simulink model "FS10"  (R2017a)
settings: Solver=VariableStepAuto  StartTime=0.0  StopTime=runtime  RelTol=1e-3
values from neighbouring files (symbols this model uses):
  C1 = [0.668571650540611,0.505734391442468,0.511990363346558,0.532740104446010,0.361957267040408,0.712570423425208,0.623515243156496,0.537105734466424,0.707123883207618,0.460578686491704]    [BaseTest.m]    (also in FStest10.m)
  C2 = [0.093600031075686,0.070802814801946,0.092158265402380,0.095893218800282,0.043434872044849,0.106885563513781,0.087292134041909,0.091307974859292,0.120211060145295,0.082904163568507]    [BaseTest.m]    (also in FStest10.m)
  dn = 0.5    [BaseTest.m]    (also in FStest10.m = 2)
  dncons = 7    [FStest10.m]
  IP = [117,104,91,78,65,52,39,26,13,0]    [BaseTest.m]    (also in FStest10.m)
  IV = 0    [BaseTest.m]    (also in FStest10.m)
  maxa = 1    [BaseTest.m]    (also in FStest10.m)
  maxv = 40    [BaseTest.m]    (also in FStest10.m)
  mina = -3    [BaseTest.m]    (also in FStest10.m)
  ring = 130    [BaseTest.m]    (also in FStest10.m)
  T = [82,96,76,78,94,117,83,100,91,111]    [BaseTest.m]    (also in FStest10.m)
  U = [0  2  2.5 3.0 3.2 3.4 3.4  4 0 0  ]    [FStest10.m]
  Ut = [0 220 240 260 280 320 400 10000 10001 10002]    [FStest10.m]
undefined symbols (not defined in the file or in its folder): DiscIntNeverNeededParam
libraries: visionstatistics x10, dspstat3 x10, powerlib_meascontrol x1
settings Model: Creator=ttal5  LastModifiedBy=ttal5

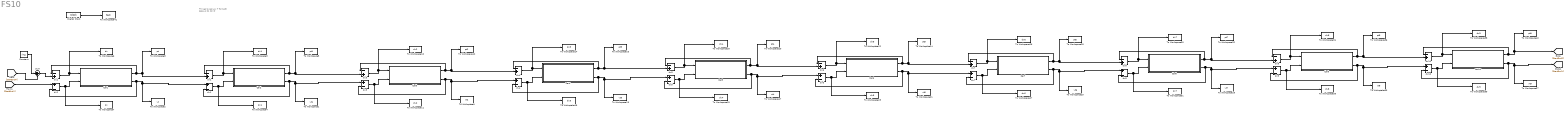
== system FS10 ==
  note: Things to set up:
      | T for both delays
      | C1
      | C2
      | IP
  Car1 : Subsystem
  Car10 : Subsystem
  Car2 : Subsystem
  Car3 : Subsystem
  Car4 : Subsystem
  Car5 : Subsystem
  Car6 : Subsystem
  Car7 : Subsystem
  Car8 : Subsystem
  Car9 : Subsystem
  Constant : Constant  Value=ring
  Digital Clock : DigitalClock  SampleTime=0.01
  Sum : Sum  Inputs=|++
  To Workspace1 : ToWorkspace  VariableName=vt1  SampleTime=0.01
  To Workspace10 : ToWorkspace  VariableName=dx2  SampleTime=0.01
  To Workspace11 : ToWorkspace  VariableName=dv2  SampleTime=0.01
  To Workspace12 : ToWorkspace  VariableName=pt2  SampleTime=0.01
  To Workspace13 : ToWorkspace  VariableName=vt3  SampleTime=0.01
  To Workspace14 : ToWorkspace  VariableName=dx3  SampleTime=0.01
  To Workspace15 : ToWorkspace  VariableName=dv3  SampleTime=0.01
  To Workspace16 : ToWorkspace  VariableName=pt3  SampleTime=0.01
  To Workspace17 : ToWorkspace  VariableName=vt4  SampleTime=0.01
  To Workspace18 : ToWorkspace  VariableName=dx4  SampleTime=0.01
  To Workspace19 : ToWorkspace  VariableName=dv4  SampleTime=0.01
  To Workspace2 : ToWorkspace  VariableName=vt  SampleTime=0.01
  To Workspace20 : ToWorkspace  VariableName=pt4  SampleTime=0.01
  To Workspace21 : ToWorkspace  VariableName=vt5  SampleTime=0.01
  To Workspace22 : ToWorkspace  VariableName=dx5  SampleTime=0.01
  To Workspace23 : ToWorkspace  VariableName=dv5  SampleTime=0.01
  To Workspace24 : ToWorkspace  VariableName=pt5  SampleTime=0.01
  To Workspace25 : ToWorkspace  VariableName=vt6  SampleTime=0.01
  To Workspace26 : ToWorkspace  VariableName=dx6  SampleTime=0.01
  To Workspace27 : ToWorkspace  VariableName=dv6  SampleTime=0.01
  To Workspace28 : ToWorkspace  VariableName=pt6  SampleTime=0.01
  To Workspace29 : ToWorkspace  VariableName=vt7  SampleTime=0.01
  To Workspace3 : ToWorkspace  VariableName=dx1  SampleTime=0.01
  To Workspace30 : ToWorkspace  VariableName=dx7  SampleTime=0.01
  To Workspace31 : ToWorkspace  VariableName=dv7  SampleTime=0.01
  To Workspace32 : ToWorkspace  VariableName=pt7  SampleTime=0.01
  To Workspace33 : ToWorkspace  VariableName=vt8  SampleTime=0.01
  To Workspace34 : ToWorkspace  VariableName=dx8  SampleTime=0.01
  To Workspace35 : ToWorkspace  VariableName=dv8  SampleTime=0.01
  To Workspace36 : ToWorkspace  VariableName=pt8  SampleTime=0.01
  To Workspace37 : ToWorkspace  VariableName=vt9  SampleTime=0.01
  To Workspace38 : ToWorkspace  VariableName=dx9  SampleTime=0.01
  To Workspace39 : ToWorkspace  VariableName=dv9  SampleTime=0.01
  To Workspace4 : ToWorkspace  VariableName=dv1  SampleTime=0.01
  To Workspace40 : ToWorkspace  VariableName=pt9  SampleTime=0.01
  To Workspace41 : ToWorkspace  VariableName=ttest  SampleTime=0.01
  To Workspace5 : ToWorkspace  VariableName=pt1  SampleTime=0.01
  To Workspace6 : ToWorkspace  VariableName=dx  SampleTime=0.01
  To Workspace7 : ToWorkspace  VariableName=dv  SampleTime=0.01
  To Workspace8 : ToWorkspace  VariableName=pt  SampleTime=0.01
  To Workspace9 : ToWorkspace  VariableName=vt2  SampleTime=0.01
  dv{1..10} (10 alike) : Sum  Inputs=+-
  dx{1..10} (10 alike) : Sum  Inputs=-+  OutMin=[0]
  wires:
  dv1/1 -> To Workspace4/1, Car2/2(dv)
  dx1/1 -> To Workspace3/1, Car2/1(dx)
  Car1/1(Pos1) -> dx2/1, dx1/2, To Workspace8/1
  Car1/2(Vel1) -> dv1/1, To Workspace2/1, dv2/2
  dv2/1 -> To Workspace7/1, Car1/2(dv)
  dx2/1 -> To Workspace6/1, Car1/1(dx)
  [StartEndP] -> Sum/2
  [StartEndV] -> dv2/1
  dv3/1 -> To Workspace11/1, Car3/2(dv)
  dx3/1 -> To Workspace10/1, Car3/1(dx)
  Car2/1(Pos1) -> dx1/1, dx3/2, To Workspace5/1
  Car2/2(Vel1) -> dv3/1, To Workspace1/1, dv1/2
  dv4/1 -> To Workspace15/1, Car4/2(dv)
  dx4/1 -> To Workspace14/1, Car4/1(dx)
  Car3/1(Pos1) -> dx3/1, dx4/2, To Workspace12/1
  Car3/2(Vel1) -> dv4/1, To Workspace9/1, dv3/2
  dv5/1 -> To Workspace19/1, Car5/2(dv)
  dx5/1 -> To Workspace18/1, Car5/1(dx)
  Car4/1(Pos1) -> dx4/1, dx5/2, To Workspace16/1
  Car4/2(Vel1) -> dv5/1, To Workspace13/1, dv4/2
  dv6/1 -> To Workspace23/1, Car6/2(dv)
  dx6/1 -> To Workspace22/1, Car6/1(dx)
  Car5/1(Pos1) -> dx5/1, dx6/2, To Workspace20/1
  Car5/2(Vel1) -> dv6/1, To Workspace17/1, dv5/2
  dv7/1 -> To Workspace27/1, Car7/2(dv)
  dx7/1 -> To Workspace26/1, Car7/1(dx)
  Car6/1(Pos1) -> dx6/1, dx7/2, To Workspace24/1
  Car6/2(Vel1) -> To Workspace21/1, dv7/1, dv6/2
  dv8/1 -> To Workspace31/1, Car8/2(dv)
  dx8/1 -> To Workspace30/1, Car8/1(dx)
  Car7/1(Pos1) -> dx7/1, dx8/2, To Workspace28/1
  Car7/2(Vel1) -> dv8/1, To Workspace25/1, dv7/2
  dv9/1 -> To Workspace35/1, Car9/2(dv)
  dx9/1 -> To Workspace34/1, Car9/1(dx)
  Car8/1(Pos1) -> dx8/1, dx9/2, To Workspace32/1
  Car8/2(Vel1) -> dv9/1, To Workspace29/1, dv8/2
  Car10/2(Vel1) -> [StartEndV], To Workspace37/1, dv10/2
  dv10/1 -> To Workspace39/1, Car10/2(dv)
  dx10/1 -> To Workspace38/1, Car10/1(dx)
  Car10/1(Pos1) -> dx10/1, [StartEndP], To Workspace40/1
  Car9/1(Pos1) -> dx9/1, dx10/2, To Workspace36/1
  Car9/2(Vel1) -> dv10/1, To Workspace33/1, dv9/2
  Constant/1 -> Sum/1
  Sum/1 -> dx2/2
  Digital Clock/1 -> To Workspace41/1

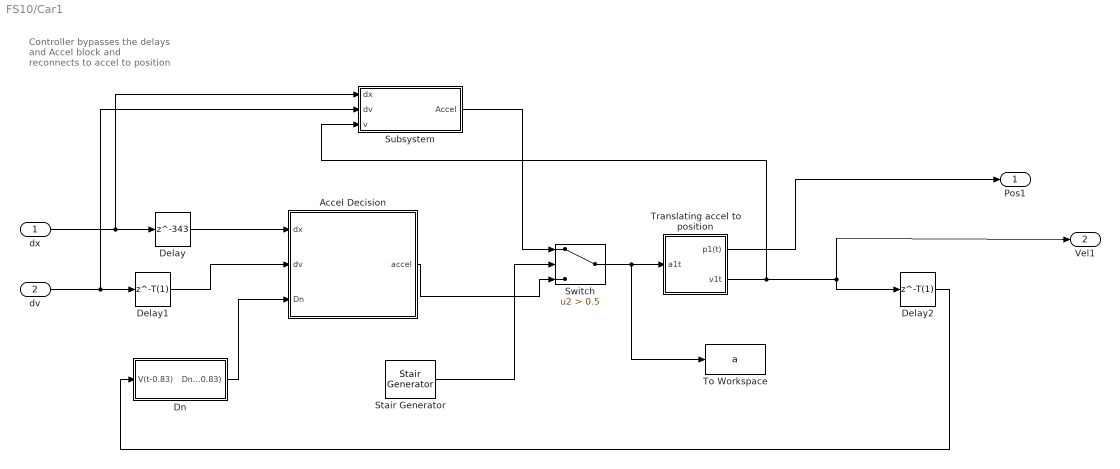
== system FS10/Car1 ==
  note: Controller bypasses the delays and Accel block and reconnects to accel to position
  dx : Inport
  dv : Inport  Port=2
  Accel Decision : Subsystem
  Delay : Delay  DelayLength=343  InitialCondition=IP(1)-IP(2)  SampleTime=0.01
  Delay1 : Delay  DelayLength=T(1)  SampleTime=0.01
  Delay2 : Delay  DelayLength=T(1)  SampleTime=0.01
  Dn : Subsystem
  Stair Generator : powerlib_meascontrol/Pulse & Signal Generators/Stair Generator  t=FStime  e=[0 1 1 0]  Ts=0.01
      settings: SourceProductName=Simscape Power Systems
  Subsystem : Subsystem
  Switch : Switch  Criteria=u2 > Threshold  Threshold=0.5
  To Workspace : ToWorkspace  VariableName=a  SampleTime=0.01
  Translating accel to position : Subsystem
  Pos1 : Outport
  Vel1 : Outport  Port=2
  wires:
  Translating accel to position/1(p1(t)) -> Pos1/1
  Delay/1 -> Accel Decision/1(dx)
  Accel Decision/1(accel) -> Switch/3
  Translating accel to position/2(v1t) -> Subsystem/3(v), Delay2/1, Vel1/1
  Delay2/1 -> Dn/1(V(t-0.83))
  Dn/1(Dn(t-0.83)) -> Accel Decision/3(Dn)
  Delay1/1 -> Accel Decision/2(dv)
  dx/1 -> Subsystem/1(dx), Delay/1
  dv/1 -> Subsystem/2("dv "), Delay1/1
  Subsystem/1(Accel) -> Switch/1
  Switch/1 -> To Workspace/1, Translating accel to position/1(a1t)
  Stair Generator/1 -> Switch/2

== system FS10/Car10 ==
  dx : Inport
  dv : Inport  Port=2
  Accel Decision : Subsystem
  Delay : Delay  DelayLength=343  InitialCondition=IP(1)-IP(2)  SampleTime=0.01
  Delay1 : Delay  DelayLength=T(10)  SampleTime=0.01
  Delay2 : Delay  DelayLength=T(10)  SampleTime=0.01
  Dn : Subsystem
  To Workspace : ToWorkspace  VariableName=a10  SampleTime=-1
  Translating accel to position : Subsystem
  Pos1 : Outport
  Vel1 : Outport  Port=2
  wires:
  Translating accel to position/1(p1(t)) -> Pos1/1
  Delay/1 -> Accel Decision/1(dx)
  Accel Decision/1(accel) -> To Workspace/1, Translating accel to position/1(a1t)
  Translating accel to position/2(v1t) -> Delay2/1, Vel1/1
  Delay2/1 -> Dn/1(V(t-0.83))
  Dn/1(Dn(t-0.83)) -> Accel Decision/3(Dn)
  Delay1/1 -> Accel Decision/2(dv)
  dx/1 -> Delay/1
  dv/1 -> Delay1/1

== system FS10/Car2 ==
  dx : Inport
  dv : Inport  Port=2
  Accel Decision : Subsystem
  Delay : Delay  DelayLength=343  InitialCondition=IP(1)-IP(2)  SampleTime=0.01
  Delay1 : Delay  DelayLength=T(2)  SampleTime=0.01
  Delay2 : Delay  DelayLength=T(2)  SampleTime=0.01
  Dn : Subsystem
  To Workspace : ToWorkspace  VariableName=a2  SampleTime=-1
  Translating accel to position : Subsystem
  Pos1 : Outport
  Vel1 : Outport  Port=2
  wires:
  Translating accel to position/1(p1(t)) -> Pos1/1
  Delay/1 -> Accel Decision/1(dx)
  Accel Decision/1(accel) -> To Workspace/1, Translating accel to position/1(a1t)
  Translating accel to position/2(v1t) -> Delay2/1, Vel1/1
  Delay2/1 -> Dn/1(V(t-0.83))
  Dn/1(Dn(t-0.83)) -> Accel Decision/3(Dn)
  Delay1/1 -> Accel Decision/2(dv)
  dx/1 -> Delay/1
  dv/1 -> Delay1/1

== system FS10/Car3 ==
  dx : Inport
  dv : Inport  Port=2
  Accel Decision : Subsystem
  Delay : Delay  DelayLength=343  InitialCondition=IP(1)-IP(2)  SampleTime=0.01
  Delay1 : Delay  DelayLength=T(3)  SampleTime=0.01
  Delay2 : Delay  DelayLength=T(3)  SampleTime=0.01
  Dn : Subsystem
  To Workspace : ToWorkspace  VariableName=a3  SampleTime=-1
  Translating accel to position : Subsystem
  Pos1 : Outport
  Vel1 : Outport  Port=2
  wires:
  Translating accel to position/1(p1(t)) -> Pos1/1
  Delay/1 -> Accel Decision/1(dx)
  Accel Decision/1(accel) -> To Workspace/1, Translating accel to position/1(a1t)
  Translating accel to position/2(v1t) -> Delay2/1, Vel1/1
  Delay2/1 -> Dn/1(V(t-0.83))
  Dn/1(Dn(t-0.83)) -> Accel Decision/3(Dn)
  Delay1/1 -> Accel Decision/2(dv)
  dx/1 -> Delay/1
  dv/1 -> Delay1/1

== system FS10/Car4 ==
  dx : Inport
  dv : Inport  Port=2
  Accel Decision : Subsystem
  Delay : Delay  DelayLength=343  InitialCondition=IP(1)-IP(2)  SampleTime=0.01
  Delay1 : Delay  DelayLength=T(4)  SampleTime=0.01
  Delay2 : Delay  DelayLength=T(4)  SampleTime=0.01
  Dn : Subsystem
  To Workspace : ToWorkspace  VariableName=a4  SampleTime=-1
  Translating accel to position : Subsystem
  Pos1 : Outport
  Vel1 : Outport  Port=2
  wires:
  Translating accel to position/1(p1(t)) -> Pos1/1
  Delay/1 -> Accel Decision/1(dx)
  Accel Decision/1(accel) -> To Workspace/1, Translating accel to position/1(a1t)
  Translating accel to position/2(v1t) -> Delay2/1, Vel1/1
  Delay2/1 -> Dn/1(V(t-0.83))
  Dn/1(Dn(t-0.83)) -> Accel Decision/3(Dn)
  Delay1/1 -> Accel Decision/2(dv)
  dx/1 -> Delay/1
  dv/1 -> Delay1/1

== system FS10/Car5 ==
  dx : Inport
  dv : Inport  Port=2
  Accel Decision : Subsystem
  Delay : Delay  DelayLength=343  InitialCondition=IP(1)-IP(2)  SampleTime=0.01
  Delay1 : Delay  DelayLength=T(5)  SampleTime=0.01
  Delay2 : Delay  DelayLength=T(5)  SampleTime=0.01
  Dn : Subsystem
  To Workspace : ToWorkspace  VariableName=a5  SampleTime=-1
  Translating accel to position : Subsystem
  Pos1 : Outport
  Vel1 : Outport  Port=2
  wires:
  Translating accel to position/1(p1(t)) -> Pos1/1
  Delay/1 -> Accel Decision/1(dx)
  Accel Decision/1(accel) -> To Workspace/1, Translating accel to position/1(a1t)
  Translating accel to position/2(v1t) -> Delay2/1, Vel1/1
  Delay2/1 -> Dn/1(V(t-0.83))
  Dn/1(Dn(t-0.83)) -> Accel Decision/3(Dn)
  Delay1/1 -> Accel Decision/2(dv)
  dx/1 -> Delay/1
  dv/1 -> Delay1/1

== system FS10/Car6 ==
  dx : Inport
  dv : Inport  Port=2
  Accel Decision : Subsystem
  Delay : Delay  DelayLength=343  InitialCondition=IP(1)-IP(2)  SampleTime=0.01
  Delay1 : Delay  DelayLength=T(6)  SampleTime=0.01
  Delay2 : Delay  DelayLength=T(6)  SampleTime=0.01
  Dn : Subsystem
  To Workspace : ToWorkspace  VariableName=a6  SampleTime=-1
  Translating accel to position : Subsystem
  Pos1 : Outport
  Vel1 : Outport  Port=2
  wires:
  Translating accel to position/1(p1(t)) -> Pos1/1
  Delay/1 -> Accel Decision/1(dx)
  Accel Decision/1(accel) -> To Workspace/1, Translating accel to position/1(a1t)
  Translating accel to position/2(v1t) -> Delay2/1, Vel1/1
  Delay2/1 -> Dn/1(V(t-0.83))
  Dn/1(Dn(t-0.83)) -> Accel Decision/3(Dn)
  Delay1/1 -> Accel Decision/2(dv)
  dx/1 -> Delay/1
  dv/1 -> Delay1/1

== system FS10/Car7 ==
  dx : Inport
  dv : Inport  Port=2
  Accel Decision : Subsystem
  Delay : Delay  DelayLength=343  InitialCondition=IP(1)-IP(2)  SampleTime=0.01
  Delay1 : Delay  DelayLength=T(7)  SampleTime=0.01
  Delay2 : Delay  DelayLength=T(7)  SampleTime=0.01
  Dn : Subsystem
  To Workspace : ToWorkspace  VariableName=a7  SampleTime=-1
  Translating accel to position : Subsystem
  Pos1 : Outport
  Vel1 : Outport  Port=2
  wires:
  Translating accel to position/1(p1(t)) -> Pos1/1
  Delay/1 -> Accel Decision/1(dx)
  Accel Decision/1(accel) -> To Workspace/1, Translating accel to position/1(a1t)
  Translating accel to position/2(v1t) -> Delay2/1, Vel1/1
  Delay2/1 -> Dn/1(V(t-0.83))
  Dn/1(Dn(t-0.83)) -> Accel Decision/3(Dn)
  Delay1/1 -> Accel Decision/2(dv)
  dx/1 -> Delay/1
  dv/1 -> Delay1/1

== system FS10/Car8 ==
  dx : Inport
  dv : Inport  Port=2
  Accel Decision : Subsystem
  Delay : Delay  DelayLength=343  InitialCondition=IP(1)-IP(2)  SampleTime=0.01
  Delay1 : Delay  DelayLength=T(8)  SampleTime=0.01
  Delay2 : Delay  DelayLength=T(8)  SampleTime=0.01
  Dn : Subsystem
  To Workspace : ToWorkspace  VariableName=a8  SampleTime=-1
  Translating accel to position : Subsystem
  Pos1 : Outport
  Vel1 : Outport  Port=2
  wires:
  Translating accel to position/1(p1(t)) -> Pos1/1
  Delay/1 -> Accel Decision/1(dx)
  Accel Decision/1(accel) -> To Workspace/1, Translating accel to position/1(a1t)
  Translating accel to position/2(v1t) -> Delay2/1, Vel1/1
  Delay2/1 -> Dn/1(V(t-0.83))
  Dn/1(Dn(t-0.83)) -> Accel Decision/3(Dn)
  Delay1/1 -> Accel Decision/2(dv)
  dx/1 -> Delay/1
  dv/1 -> Delay1/1

== system FS10/Car9 ==
  dx : Inport
  dv : Inport  Port=2
  Accel Decision : Subsystem
  Delay : Delay  DelayLength=343  InitialCondition=IP(1)-IP(2)  SampleTime=0.01
  Delay1 : Delay  DelayLength=T(9)  SampleTime=0.01
  Delay2 : Delay  DelayLength=T(9)  SampleTime=0.01
  Dn : Subsystem
  To Workspace : ToWorkspace  VariableName=a9  SampleTime=-1
  Translating accel to position : Subsystem
  Pos1 : Outport
  Vel1 : Outport  Port=2
  wires:
  Translating accel to position/1(p1(t)) -> Pos1/1
  Delay/1 -> Accel Decision/1(dx)
  Accel Decision/1(accel) -> To Workspace/1, Translating accel to position/1(a1t)
  Translating accel to position/2(v1t) -> Delay2/1, Vel1/1
  Delay2/1 -> Dn/1(V(t-0.83))
  Dn/1(Dn(t-0.83)) -> Accel Decision/3(Dn)
  Delay1/1 -> Accel Decision/2(dv)
  dx/1 -> Delay/1
  dv/1 -> Delay1/1

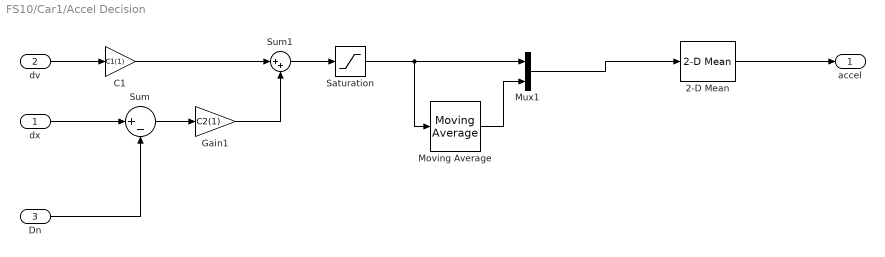
== system FS10/Car1/Accel Decision ==
  dx : Inport
  dv : Inport  Port=2
  Dn : Inport  Port=3
  2-D Mean : visionstatistics/2-D Mean  run=off  reset_popup=None  directionMode=Entire input  dimension=1  treatSBRowAsCol=on  roiEnable=off  roiType=Rectangles  roiPortion=Entire ROI  roiOutput=Individual statistics for each ROI  roiFlag=off  outputDataTypeStr=Inherit: Same as accumulator  outputLastDataTypeStr=Inherit: Same as accumulator  outputMin=[]  outputMax=[]  accumMode=Binary point scaling  accumWordLength=32  accumFracLength=0  accumDataTypeStr=fixdt([],32,0)  accumLastDataTypeStr=fixdt([],32,0)  roundingMode=Floor  overflowMode=off
      settings: SourceProductName=Computer Vision System Toolbox  SourceProductBaseCode=VP
  C1 : Gain  Gain=C1(1)
  Gain1 : Gain  Gain=C2(1)
  Moving Average : dspstat3/Moving Average  Method=Sliding window  SpecifyWindowLength=on  WindowLength=ave  ForgettingFactor=0.9  SimulateUsing=Code generation
  Mux1 : Mux  Inputs=2
  Saturation : Saturate  UpperLimit=maxa  LowerLimit=mina
  Sum : Sum  Inputs=|+-
  Sum1 : Sum  Inputs=|++  OutMax=[3]
  accel : Outport  OutMax=[3]  SampleTime=0.01
  wires:
  dv/1 -> C1/1
  dx/1 -> Sum/1
  Sum/1 -> Gain1/1
  C1/1 -> Sum1/1
  Gain1/1 -> Sum1/2
  Sum1/1 -> Saturation/1
  Dn/1 -> Sum/2
  Moving Average/1 -> Mux1/2
  Mux1/1 -> 2-D Mean/1
  Saturation/1 -> Moving Average/1, Mux1/1
  2-D Mean/1 -> accel/1

== system FS10/Car1/Dn ==
  V(t-0.83) : Inport
  0.5v : Gain  Gain=dn
  Constant : Constant  Value=dncons
  Sum : Sum  Inputs=|++
  Dn(t-0.83) : Outport
  wires:
  V(t-0.83)/1 -> 0.5v/1
  0.5v/1 -> Sum/1
  Constant/1 -> Sum/2
  Sum/1 -> Dn(t-0.83)/1

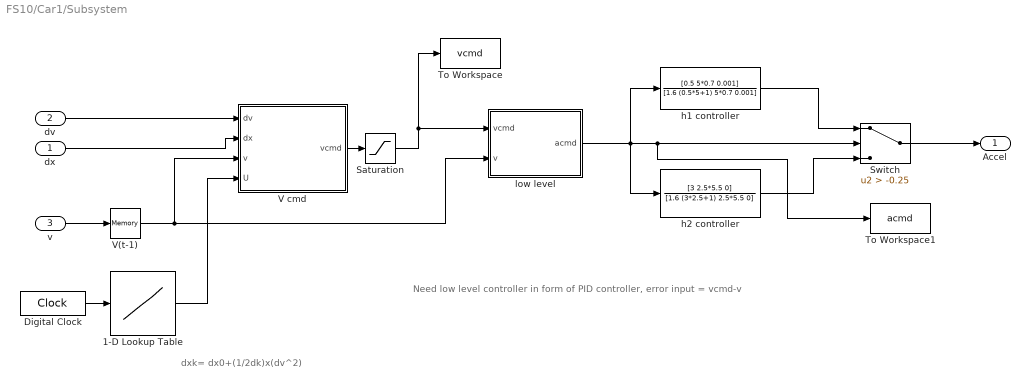
== system FS10/Car1/Subsystem ==
  note: Need low level controller in form of PID controller, error input = vcmd-v
  note: dxk= dx0+(1/2dk)x(dv^2)
  dx : Inport
  "dv " : Inport  Port=2
  v : Inport  Port=3
  1-D Lookup Table : Lookup_n-D  NumberOfTableDimensions=1  BreakpointsForDimension1=Ut  Table=U  InternalRulePriority=Speed  RndMeth=Simplest  InputSameDT=on
  Digital Clock : DigitalClock  SampleTime=0.01
  Saturation : Saturate  UpperLimit=maxv  LowerLimit=0
  Switch : Switch  Criteria=u2 > Threshold  Threshold=-0.25
  To Workspace : ToWorkspace  VariableName=vcmd  SampleTime=0.01
  To Workspace1 : ToWorkspace  VariableName=acmd  SampleTime=0.01
  V cmd : MATLAB Function  TreatAsAtomicUnit=on
  V(t-1) : Memory
  h1 controller : TransferFcn  Numerator=[0.5 5*0.7 0.001]  Denominator=[1.6 (0.5*5+1) 5*0.7 0.001]
  h2 controller : TransferFcn  Numerator=[3 2.5*5.5 0]  Denominator=[1.6 (3*2.5+1) 2.5*5.5 0]
  low level : MATLAB Function  TreatAsAtomicUnit=on
  Accel : Outport
  wires:
  "dv "/1 -> V cmd/1(dv)
  dx/1 -> V cmd/2(dx)
  v/1 -> V(t-1)/1
  V(t-1)/1 -> low level/2(v), V cmd/3(v)
  1-D Lookup Table/1 -> V cmd/4(U)
  Digital Clock/1 -> 1-D Lookup Table/1
  h1 controller/1 -> Switch/1
  h2 controller/1 -> Switch/3
  V cmd/1(vcmd) -> Saturation/1
  Saturation/1 -> To Workspace/1, low level/1(vcmd)
  Switch/1 -> Accel/1
  low level/1(acmd) -> h2 controller/1, h1 controller/1, To Workspace1/1, Switch/2

== system FS10/Car1/Translating accel to position ==
  a1t : Inport
  Discrete-Time Integrator : DiscreteIntegrator  InitialCondition=IV  InitialConditionSetting=State (most efficient)  SampleTime=-1  OutMin=0  OutMax=maxv  LimitOutput=on  UpperSaturationLimit=maxv  LowerSaturationLimit=0  ICPrevOutput=DiscIntNeverNeededParam  ICPrevScaledInput=DiscIntNeverNeededParam
  Discrete-Time Integrator1 : DiscreteIntegrator  InitialCondition=IP(1)  InitialConditionSetting=State (most efficient)  SampleTime=-1  ICPrevOutput=DiscIntNeverNeededParam  ICPrevScaledInput=DiscIntNeverNeededParam
  p1(t) : Outport
  v1t : Outport  Port=2
  wires:
  a1t/1 -> Discrete-Time Integrator/1
  Discrete-Time Integrator1/1 -> p1(t)/1
  Discrete-Time Integrator/1 -> Discrete-Time Integrator1/1, v1t/1

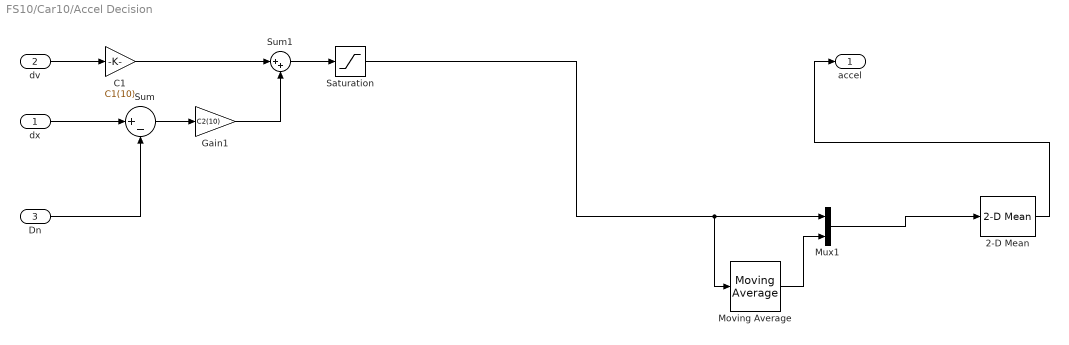
== system FS10/Car10/Accel Decision ==
  dx : Inport
  dv : Inport  Port=2
  Dn : Inport  Port=3
  2-D Mean : visionstatistics/2-D Mean  run=off  reset_popup=None  directionMode=Entire input  dimension=1  treatSBRowAsCol=on  roiEnable=off  roiType=Rectangles  roiPortion=Entire ROI  roiOutput=Individual statistics for each ROI  roiFlag=off  outputDataTypeStr=Inherit: Same as accumulator  outputLastDataTypeStr=Inherit: Same as accumulator  outputMin=[]  outputMax=[]  accumMode=Binary point scaling  accumWordLength=32  accumFracLength=0  accumDataTypeStr=fixdt([],32,0)  accumLastDataTypeStr=fixdt([],32,0)  roundingMode=Floor  overflowMode=off
      settings: SourceProductName=Computer Vision System Toolbox  SourceProductBaseCode=VP
  C1 : Gain  Gain=C1(10)
  Gain1 : Gain  Gain=C2(10)
  Moving Average : dspstat3/Moving Average  Method=Sliding window  SpecifyWindowLength=on  WindowLength=ave  ForgettingFactor=0.9  SimulateUsing=Code generation
  Mux1 : Mux  Inputs=2
  Saturation : Saturate  UpperLimit=maxa  LowerLimit=mina
  Sum : Sum  Inputs=|+-
  Sum1 : Sum  Inputs=|++  OutMax=[3]
  accel : Outport  OutMax=[3]  SampleTime=0.01
  wires:
  dv/1 -> C1/1
  dx/1 -> Sum/1
  Sum/1 -> Gain1/1
  C1/1 -> Sum1/1
  Gain1/1 -> Sum1/2
  Sum1/1 -> Saturation/1
  Dn/1 -> Sum/2
  Moving Average/1 -> Mux1/2
  Mux1/1 -> 2-D Mean/1
  Saturation/1 -> Moving Average/1, Mux1/1
  2-D Mean/1 -> accel/1

== system FS10/Car10/Dn ==
  V(t-0.83) : Inport
  0.5v : Gain  Gain=dn
  Constant : Constant  Value=dncons
  Sum : Sum  Inputs=|++
  Dn(t-0.83) : Outport
  wires:
  V(t-0.83)/1 -> 0.5v/1
  0.5v/1 -> Sum/1
  Constant/1 -> Sum/2
  Sum/1 -> Dn(t-0.83)/1

== system FS10/Car10/Translating accel to position ==
  a1t : Inport
  Discrete-Time Integrator : DiscreteIntegrator  InitialCondition=IV  InitialConditionSetting=State (most efficient)  SampleTime=-1  OutMin=0  OutMax=maxv  LimitOutput=on  UpperSaturationLimit=maxv  LowerSaturationLimit=0  ICPrevOutput=DiscIntNeverNeededParam  ICPrevScaledInput=DiscIntNeverNeededParam
  Discrete-Time Integrator1 : DiscreteIntegrator  InitialCondition=IP(10)  InitialConditionSetting=State (most efficient)  SampleTime=-1  ICPrevOutput=DiscIntNeverNeededParam  ICPrevScaledInput=DiscIntNeverNeededParam
  p1(t) : Outport
  v1t : Outport  Port=2
  wires:
  a1t/1 -> Discrete-Time Integrator/1
  Discrete-Time Integrator1/1 -> p1(t)/1
  Discrete-Time Integrator/1 -> Discrete-Time Integrator1/1, v1t/1

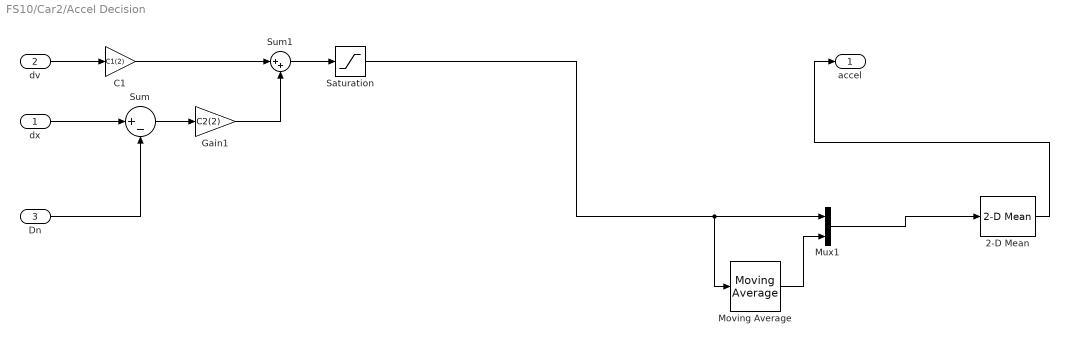
== system FS10/Car2/Accel Decision ==
  dx : Inport
  dv : Inport  Port=2
  Dn : Inport  Port=3
  2-D Mean : visionstatistics/2-D Mean  run=off  reset_popup=None  directionMode=Entire input  dimension=1  treatSBRowAsCol=on  roiEnable=off  roiType=Rectangles  roiPortion=Entire ROI  roiOutput=Individual statistics for each ROI  roiFlag=off  outputDataTypeStr=Inherit: Same as accumulator  outputLastDataTypeStr=Inherit: Same as accumulator  outputMin=[]  outputMax=[]  accumMode=Binary point scaling  accumWordLength=32  accumFracLength=0  accumDataTypeStr=fixdt([],32,0)  accumLastDataTypeStr=fixdt([],32,0)  roundingMode=Floor  overflowMode=off
      settings: SourceProductName=Computer Vision System Toolbox  SourceProductBaseCode=VP
  C1 : Gain  Gain=C1(2)
  Gain1 : Gain  Gain=C2(2)
  Moving Average : dspstat3/Moving Average  Method=Sliding window  SpecifyWindowLength=on  WindowLength=ave  ForgettingFactor=0.9  SimulateUsing=Code generation
  Mux1 : Mux  Inputs=2
  Saturation : Saturate  UpperLimit=maxa  LowerLimit=mina
  Sum : Sum  Inputs=|+-
  Sum1 : Sum  Inputs=|++  OutMax=[3]
  accel : Outport  OutMax=[3]  SampleTime=0.01
  wires:
  dv/1 -> C1/1
  dx/1 -> Sum/1
  Sum/1 -> Gain1/1
  C1/1 -> Sum1/1
  Gain1/1 -> Sum1/2
  Sum1/1 -> Saturation/1
  Dn/1 -> Sum/2
  Moving Average/1 -> Mux1/2
  Mux1/1 -> 2-D Mean/1
  Saturation/1 -> Moving Average/1, Mux1/1
  2-D Mean/1 -> accel/1

== system FS10/Car2/Dn ==
  V(t-0.83) : Inport
  0.5v : Gain  Gain=dn
  Constant : Constant  Value=dncons
  Sum : Sum  Inputs=|++
  Dn(t-0.83) : Outport
  wires:
  V(t-0.83)/1 -> 0.5v/1
  0.5v/1 -> Sum/1
  Constant/1 -> Sum/2
  Sum/1 -> Dn(t-0.83)/1

== system FS10/Car2/Translating accel to position ==
  a1t : Inport
  Discrete-Time Integrator : DiscreteIntegrator  InitialCondition=IV  InitialConditionSetting=State (most efficient)  SampleTime=-1  OutMin=0  OutMax=maxv  LimitOutput=on  UpperSaturationLimit=maxv  LowerSaturationLimit=0  ICPrevOutput=DiscIntNeverNeededParam  ICPrevScaledInput=DiscIntNeverNeededParam
  Discrete-Time Integrator1 : DiscreteIntegrator  InitialCondition=IP(2)  InitialConditionSetting=State (most efficient)  SampleTime=-1  ICPrevOutput=DiscIntNeverNeededParam  ICPrevScaledInput=DiscIntNeverNeededParam
  p1(t) : Outport
  v1t : Outport  Port=2
  wires:
  a1t/1 -> Discrete-Time Integrator/1
  Discrete-Time Integrator1/1 -> p1(t)/1
  Discrete-Time Integrator/1 -> Discrete-Time Integrator1/1, v1t/1

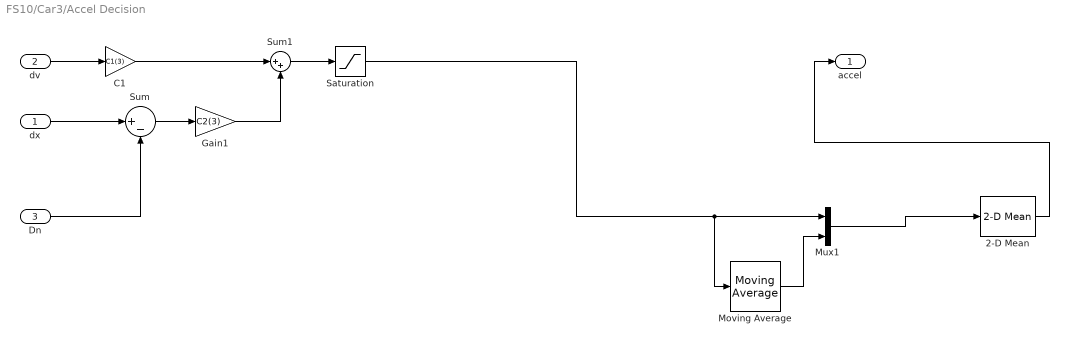
== system FS10/Car3/Accel Decision ==
  dx : Inport
  dv : Inport  Port=2
  Dn : Inport  Port=3
  2-D Mean : visionstatistics/2-D Mean  run=off  reset_popup=None  directionMode=Entire input  dimension=1  treatSBRowAsCol=on  roiEnable=off  roiType=Rectangles  roiPortion=Entire ROI  roiOutput=Individual statistics for each ROI  roiFlag=off  outputDataTypeStr=Inherit: Same as accumulator  outputLastDataTypeStr=Inherit: Same as accumulator  outputMin=[]  outputMax=[]  accumMode=Binary point scaling  accumWordLength=32  accumFracLength=0  accumDataTypeStr=fixdt([],32,0)  accumLastDataTypeStr=fixdt([],32,0)  roundingMode=Floor  overflowMode=off
      settings: SourceProductName=Computer Vision System Toolbox  SourceProductBaseCode=VP
  C1 : Gain  Gain=C1(3)
  Gain1 : Gain  Gain=C2(3)
  Moving Average : dspstat3/Moving Average  Method=Sliding window  SpecifyWindowLength=on  WindowLength=ave  ForgettingFactor=0.9  SimulateUsing=Code generation
  Mux1 : Mux  Inputs=2
  Saturation : Saturate  UpperLimit=maxa  LowerLimit=mina
  Sum : Sum  Inputs=|+-
  Sum1 : Sum  Inputs=|++  OutMax=[3]
  accel : Outport  OutMax=[3]  SampleTime=0.01
  wires:
  dv/1 -> C1/1
  dx/1 -> Sum/1
  Sum/1 -> Gain1/1
  C1/1 -> Sum1/1
  Gain1/1 -> Sum1/2
  Sum1/1 -> Saturation/1
  Dn/1 -> Sum/2
  Moving Average/1 -> Mux1/2
  Mux1/1 -> 2-D Mean/1
  Saturation/1 -> Moving Average/1, Mux1/1
  2-D Mean/1 -> accel/1

== system FS10/Car3/Dn ==
  V(t-0.83) : Inport
  0.5v : Gain  Gain=dn
  Constant : Constant  Value=dncons
  Sum : Sum  Inputs=|++
  Dn(t-0.83) : Outport
  wires:
  V(t-0.83)/1 -> 0.5v/1
  0.5v/1 -> Sum/1
  Constant/1 -> Sum/2
  Sum/1 -> Dn(t-0.83)/1

== system FS10/Car3/Translating accel to position ==
  a1t : Inport
  Discrete-Time Integrator : DiscreteIntegrator  InitialCondition=IV  InitialConditionSetting=State (most efficient)  SampleTime=-1  OutMin=0  OutMax=maxv  LimitOutput=on  UpperSaturationLimit=maxv  LowerSaturationLimit=0  ICPrevOutput=DiscIntNeverNeededParam  ICPrevScaledInput=DiscIntNeverNeededParam
  Discrete-Time Integrator1 : DiscreteIntegrator  InitialCondition=IP(3)  InitialConditionSetting=State (most efficient)  SampleTime=-1  ICPrevOutput=DiscIntNeverNeededParam  ICPrevScaledInput=DiscIntNeverNeededParam
  p1(t) : Outport
  v1t : Outport  Port=2
  wires:
  a1t/1 -> Discrete-Time Integrator/1
  Discrete-Time Integrator1/1 -> p1(t)/1
  Discrete-Time Integrator/1 -> Discrete-Time Integrator1/1, v1t/1

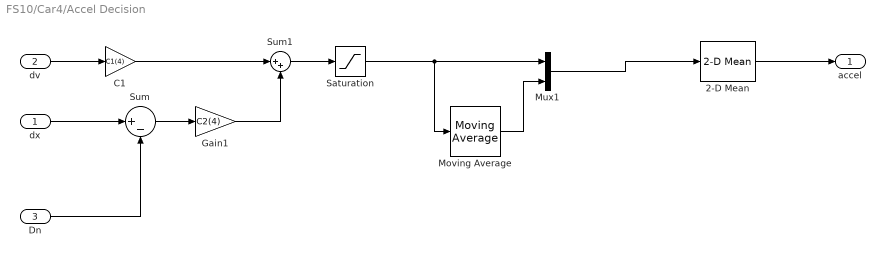
== system FS10/Car4/Accel Decision ==
  dx : Inport
  dv : Inport  Port=2
  Dn : Inport  Port=3
  2-D Mean : visionstatistics/2-D Mean  run=off  reset_popup=None  directionMode=Entire input  dimension=1  treatSBRowAsCol=on  roiEnable=off  roiType=Rectangles  roiPortion=Entire ROI  roiOutput=Individual statistics for each ROI  roiFlag=off  outputDataTypeStr=Inherit: Same as accumulator  outputLastDataTypeStr=Inherit: Same as accumulator  outputMin=[]  outputMax=[]  accumMode=Binary point scaling  accumWordLength=32  accumFracLength=0  accumDataTypeStr=fixdt([],32,0)  accumLastDataTypeStr=fixdt([],32,0)  roundingMode=Floor  overflowMode=off
      settings: SourceProductName=Computer Vision System Toolbox  SourceProductBaseCode=VP
  C1 : Gain  Gain=C1(4)
  Gain1 : Gain  Gain=C2(4)
  Moving Average : dspstat3/Moving Average  Method=Sliding window  SpecifyWindowLength=on  WindowLength=ave  ForgettingFactor=0.9  SimulateUsing=Code generation
  Mux1 : Mux  Inputs=2
  Saturation : Saturate  UpperLimit=maxa  LowerLimit=mina
  Sum : Sum  Inputs=|+-
  Sum1 : Sum  Inputs=|++  OutMax=[3]
  accel : Outport  OutMax=[3]  SampleTime=0.01
  wires:
  dv/1 -> C1/1
  dx/1 -> Sum/1
  Sum/1 -> Gain1/1
  C1/1 -> Sum1/1
  Gain1/1 -> Sum1/2
  Sum1/1 -> Saturation/1
  Dn/1 -> Sum/2
  Moving Average/1 -> Mux1/2
  Mux1/1 -> 2-D Mean/1
  Saturation/1 -> Moving Average/1, Mux1/1
  2-D Mean/1 -> accel/1

== system FS10/Car4/Dn ==
  V(t-0.83) : Inport
  0.5v : Gain  Gain=dn
  Constant : Constant  Value=dncons
  Sum : Sum  Inputs=|++
  Dn(t-0.83) : Outport
  wires:
  V(t-0.83)/1 -> 0.5v/1
  0.5v/1 -> Sum/1
  Constant/1 -> Sum/2
  Sum/1 -> Dn(t-0.83)/1

== system FS10/Car4/Translating accel to position ==
  a1t : Inport
  Discrete-Time Integrator : DiscreteIntegrator  InitialCondition=IV  InitialConditionSetting=State (most efficient)  SampleTime=-1  OutMin=0  OutMax=maxv  LimitOutput=on  UpperSaturationLimit=maxv  LowerSaturationLimit=0  ICPrevOutput=DiscIntNeverNeededParam  ICPrevScaledInput=DiscIntNeverNeededParam
  Discrete-Time Integrator1 : DiscreteIntegrator  InitialCondition=IP(4)  InitialConditionSetting=State (most efficient)  SampleTime=-1  ICPrevOutput=DiscIntNeverNeededParam  ICPrevScaledInput=DiscIntNeverNeededParam
  p1(t) : Outport
  v1t : Outport  Port=2
  wires:
  a1t/1 -> Discrete-Time Integrator/1
  Discrete-Time Integrator1/1 -> p1(t)/1
  Discrete-Time Integrator/1 -> Discrete-Time Integrator1/1, v1t/1

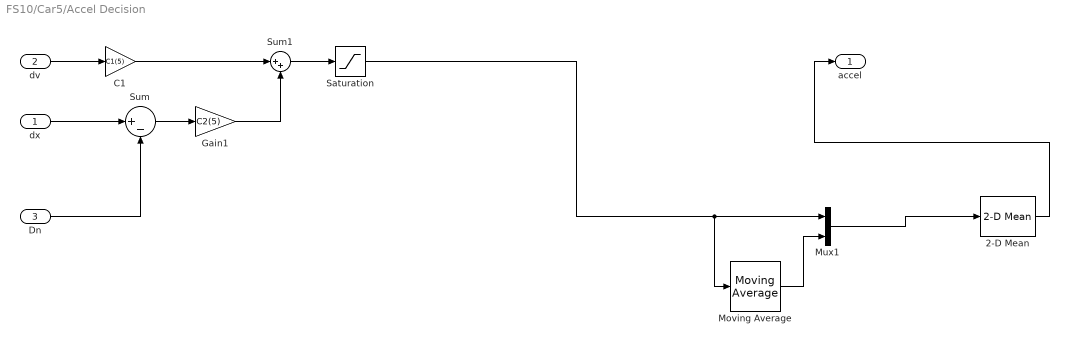
== system FS10/Car5/Accel Decision ==
  dx : Inport
  dv : Inport  Port=2
  Dn : Inport  Port=3
  2-D Mean : visionstatistics/2-D Mean  run=off  reset_popup=None  directionMode=Entire input  dimension=1  treatSBRowAsCol=on  roiEnable=off  roiType=Rectangles  roiPortion=Entire ROI  roiOutput=Individual statistics for each ROI  roiFlag=off  outputDataTypeStr=Inherit: Same as accumulator  outputLastDataTypeStr=Inherit: Same as accumulator  outputMin=[]  outputMax=[]  accumMode=Binary point scaling  accumWordLength=32  accumFracLength=0  accumDataTypeStr=fixdt([],32,0)  accumLastDataTypeStr=fixdt([],32,0)  roundingMode=Floor  overflowMode=off
      settings: SourceProductName=Computer Vision System Toolbox  SourceProductBaseCode=VP
  C1 : Gain  Gain=C1(5)
  Gain1 : Gain  Gain=C2(5)
  Moving Average : dspstat3/Moving Average  Method=Sliding window  SpecifyWindowLength=on  WindowLength=ave  ForgettingFactor=0.9  SimulateUsing=Code generation
  Mux1 : Mux  Inputs=2
  Saturation : Saturate  UpperLimit=maxa  LowerLimit=mina
  Sum : Sum  Inputs=|+-
  Sum1 : Sum  Inputs=|++  OutMax=[3]
  accel : Outport  OutMax=[3]  SampleTime=0.01
  wires:
  dv/1 -> C1/1
  dx/1 -> Sum/1
  Sum/1 -> Gain1/1
  C1/1 -> Sum1/1
  Gain1/1 -> Sum1/2
  Sum1/1 -> Saturation/1
  Dn/1 -> Sum/2
  Moving Average/1 -> Mux1/2
  Mux1/1 -> 2-D Mean/1
  Saturation/1 -> Moving Average/1, Mux1/1
  2-D Mean/1 -> accel/1

== system FS10/Car5/Dn ==
  V(t-0.83) : Inport
  0.5v : Gain  Gain=dn
  Constant : Constant  Value=dncons
  Sum : Sum  Inputs=|++
  Dn(t-0.83) : Outport
  wires:
  V(t-0.83)/1 -> 0.5v/1
  0.5v/1 -> Sum/1
  Constant/1 -> Sum/2
  Sum/1 -> Dn(t-0.83)/1

== system FS10/Car5/Translating accel to position ==
  a1t : Inport
  Discrete-Time Integrator : DiscreteIntegrator  InitialCondition=IV  InitialConditionSetting=State (most efficient)  SampleTime=-1  OutMin=0  OutMax=maxv  LimitOutput=on  UpperSaturationLimit=maxv  LowerSaturationLimit=0  ICPrevOutput=DiscIntNeverNeededParam  ICPrevScaledInput=DiscIntNeverNeededParam
  Discrete-Time Integrator1 : DiscreteIntegrator  InitialCondition=IP(5)  InitialConditionSetting=State (most efficient)  SampleTime=-1  ICPrevOutput=DiscIntNeverNeededParam  ICPrevScaledInput=DiscIntNeverNeededParam
  p1(t) : Outport
  v1t : Outport  Port=2
  wires:
  a1t/1 -> Discrete-Time Integrator/1
  Discrete-Time Integrator1/1 -> p1(t)/1
  Discrete-Time Integrator/1 -> Discrete-Time Integrator1/1, v1t/1

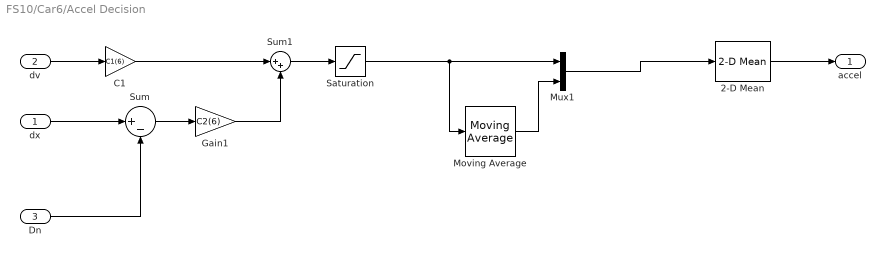
== system FS10/Car6/Accel Decision ==
  dx : Inport
  dv : Inport  Port=2
  Dn : Inport  Port=3
  2-D Mean : visionstatistics/2-D Mean  run=off  reset_popup=None  directionMode=Entire input  dimension=1  treatSBRowAsCol=on  roiEnable=off  roiType=Rectangles  roiPortion=Entire ROI  roiOutput=Individual statistics for each ROI  roiFlag=off  outputDataTypeStr=Inherit: Same as accumulator  outputLastDataTypeStr=Inherit: Same as accumulator  outputMin=[]  outputMax=[]  accumMode=Binary point scaling  accumWordLength=32  accumFracLength=0  accumDataTypeStr=fixdt([],32,0)  accumLastDataTypeStr=fixdt([],32,0)  roundingMode=Floor  overflowMode=off
      settings: SourceProductName=Computer Vision System Toolbox  SourceProductBaseCode=VP
  C1 : Gain  Gain=C1(6)
  Gain1 : Gain  Gain=C2(6)
  Moving Average : dspstat3/Moving Average  Method=Sliding window  SpecifyWindowLength=on  WindowLength=ave  ForgettingFactor=0.9  SimulateUsing=Code generation
  Mux1 : Mux  Inputs=2
  Saturation : Saturate  UpperLimit=maxa  LowerLimit=mina
  Sum : Sum  Inputs=|+-
  Sum1 : Sum  Inputs=|++  OutMax=[3]
  accel : Outport  OutMax=[3]  SampleTime=0.01
  wires:
  dv/1 -> C1/1
  dx/1 -> Sum/1
  Sum/1 -> Gain1/1
  C1/1 -> Sum1/1
  Gain1/1 -> Sum1/2
  Sum1/1 -> Saturation/1
  Dn/1 -> Sum/2
  Moving Average/1 -> Mux1/2
  Mux1/1 -> 2-D Mean/1
  Saturation/1 -> Moving Average/1, Mux1/1
  2-D Mean/1 -> accel/1

== system FS10/Car6/Dn ==
  V(t-0.83) : Inport
  0.5v : Gain  Gain=dn
  Constant : Constant  Value=dncons
  Sum : Sum  Inputs=|++
  Dn(t-0.83) : Outport
  wires:
  V(t-0.83)/1 -> 0.5v/1
  0.5v/1 -> Sum/1
  Constant/1 -> Sum/2
  Sum/1 -> Dn(t-0.83)/1

== system FS10/Car6/Translating accel to position ==
  a1t : Inport
  Discrete-Time Integrator : DiscreteIntegrator  InitialCondition=IV  InitialConditionSetting=State (most efficient)  SampleTime=-1  OutMin=0  OutMax=maxv  LimitOutput=on  UpperSaturationLimit=maxv  LowerSaturationLimit=0  ICPrevOutput=DiscIntNeverNeededParam  ICPrevScaledInput=DiscIntNeverNeededParam
  Discrete-Time Integrator1 : DiscreteIntegrator  InitialCondition=IP(6)  InitialConditionSetting=State (most efficient)  SampleTime=-1  ICPrevOutput=DiscIntNeverNeededParam  ICPrevScaledInput=DiscIntNeverNeededParam
  p1(t) : Outport
  v1t : Outport  Port=2
  wires:
  a1t/1 -> Discrete-Time Integrator/1
  Discrete-Time Integrator1/1 -> p1(t)/1
  Discrete-Time Integrator/1 -> Discrete-Time Integrator1/1, v1t/1

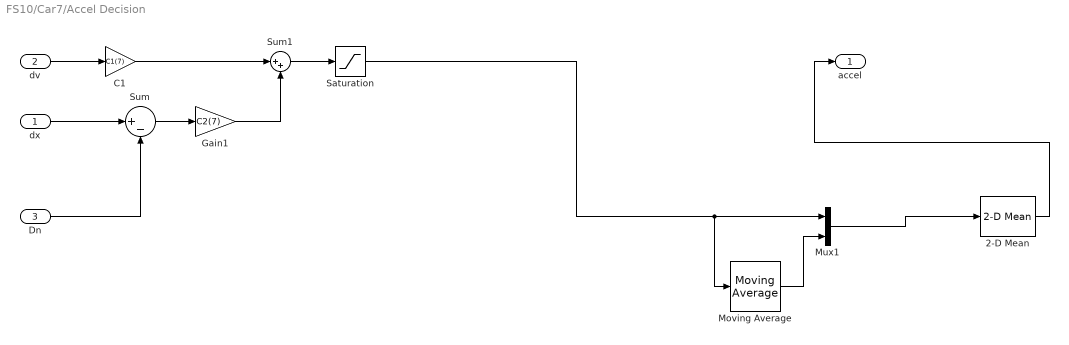
== system FS10/Car7/Accel Decision ==
  dx : Inport
  dv : Inport  Port=2
  Dn : Inport  Port=3
  2-D Mean : visionstatistics/2-D Mean  run=off  reset_popup=None  directionMode=Entire input  dimension=1  treatSBRowAsCol=on  roiEnable=off  roiType=Rectangles  roiPortion=Entire ROI  roiOutput=Individual statistics for each ROI  roiFlag=off  outputDataTypeStr=Inherit: Same as accumulator  outputLastDataTypeStr=Inherit: Same as accumulator  outputMin=[]  outputMax=[]  accumMode=Binary point scaling  accumWordLength=32  accumFracLength=0  accumDataTypeStr=fixdt([],32,0)  accumLastDataTypeStr=fixdt([],32,0)  roundingMode=Floor  overflowMode=off
      settings: SourceProductName=Computer Vision System Toolbox  SourceProductBaseCode=VP
  C1 : Gain  Gain=C1(7)
  Gain1 : Gain  Gain=C2(7)
  Moving Average : dspstat3/Moving Average  Method=Sliding window  SpecifyWindowLength=on  WindowLength=ave  ForgettingFactor=0.9  SimulateUsing=Code generation
  Mux1 : Mux  Inputs=2
  Saturation : Saturate  UpperLimit=maxa  LowerLimit=mina
  Sum : Sum  Inputs=|+-
  Sum1 : Sum  Inputs=|++  OutMax=[3]
  accel : Outport  OutMax=[3]  SampleTime=0.01
  wires:
  dv/1 -> C1/1
  dx/1 -> Sum/1
  Sum/1 -> Gain1/1
  C1/1 -> Sum1/1
  Gain1/1 -> Sum1/2
  Sum1/1 -> Saturation/1
  Dn/1 -> Sum/2
  Moving Average/1 -> Mux1/2
  Mux1/1 -> 2-D Mean/1
  Saturation/1 -> Moving Average/1, Mux1/1
  2-D Mean/1 -> accel/1

== system FS10/Car7/Dn ==
  V(t-0.83) : Inport
  0.5v : Gain  Gain=dn
  Constant : Constant  Value=dncons
  Sum : Sum  Inputs=|++
  Dn(t-0.83) : Outport
  wires:
  V(t-0.83)/1 -> 0.5v/1
  0.5v/1 -> Sum/1
  Constant/1 -> Sum/2
  Sum/1 -> Dn(t-0.83)/1

== system FS10/Car7/Translating accel to position ==
  a1t : Inport
  Discrete-Time Integrator : DiscreteIntegrator  InitialCondition=IV  InitialConditionSetting=State (most efficient)  SampleTime=-1  OutMin=0  OutMax=maxv  LimitOutput=on  UpperSaturationLimit=maxv  LowerSaturationLimit=0  ICPrevOutput=DiscIntNeverNeededParam  ICPrevScaledInput=DiscIntNeverNeededParam
  Discrete-Time Integrator1 : DiscreteIntegrator  InitialCondition=IP(7)  InitialConditionSetting=State (most efficient)  SampleTime=-1  ICPrevOutput=DiscIntNeverNeededParam  ICPrevScaledInput=DiscIntNeverNeededParam
  p1(t) : Outport
  v1t : Outport  Port=2
  wires:
  a1t/1 -> Discrete-Time Integrator/1
  Discrete-Time Integrator1/1 -> p1(t)/1
  Discrete-Time Integrator/1 -> Discrete-Time Integrator1/1, v1t/1

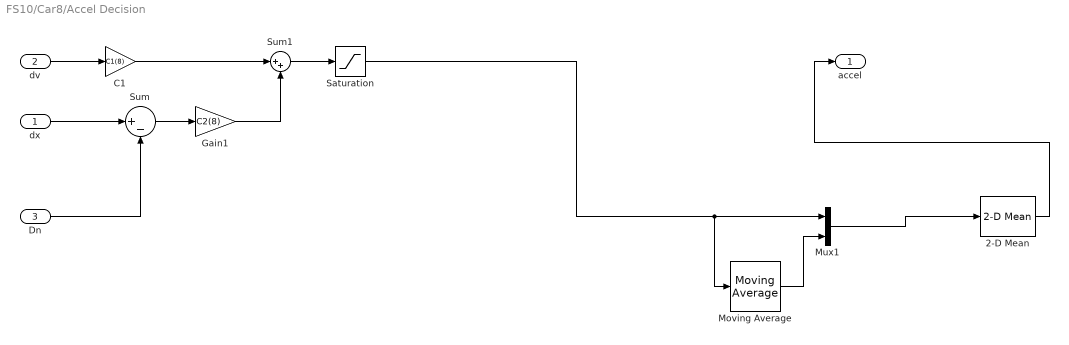
== system FS10/Car8/Accel Decision ==
  dx : Inport
  dv : Inport  Port=2
  Dn : Inport  Port=3
  2-D Mean : visionstatistics/2-D Mean  run=off  reset_popup=None  directionMode=Entire input  dimension=1  treatSBRowAsCol=on  roiEnable=off  roiType=Rectangles  roiPortion=Entire ROI  roiOutput=Individual statistics for each ROI  roiFlag=off  outputDataTypeStr=Inherit: Same as accumulator  outputLastDataTypeStr=Inherit: Same as accumulator  outputMin=[]  outputMax=[]  accumMode=Binary point scaling  accumWordLength=32  accumFracLength=0  accumDataTypeStr=fixdt([],32,0)  accumLastDataTypeStr=fixdt([],32,0)  roundingMode=Floor  overflowMode=off
      settings: SourceProductName=Computer Vision System Toolbox  SourceProductBaseCode=VP
  C1 : Gain  Gain=C1(8)
  Gain1 : Gain  Gain=C2(8)
  Moving Average : dspstat3/Moving Average  Method=Sliding window  SpecifyWindowLength=on  WindowLength=ave  ForgettingFactor=0.9  SimulateUsing=Code generation
  Mux1 : Mux  Inputs=2
  Saturation : Saturate  UpperLimit=maxa  LowerLimit=mina
  Sum : Sum  Inputs=|+-
  Sum1 : Sum  Inputs=|++  OutMax=[3]
  accel : Outport  OutMax=[3]  SampleTime=0.01
  wires:
  dv/1 -> C1/1
  dx/1 -> Sum/1
  Sum/1 -> Gain1/1
  C1/1 -> Sum1/1
  Gain1/1 -> Sum1/2
  Sum1/1 -> Saturation/1
  Dn/1 -> Sum/2
  Moving Average/1 -> Mux1/2
  Mux1/1 -> 2-D Mean/1
  Saturation/1 -> Moving Average/1, Mux1/1
  2-D Mean/1 -> accel/1

== system FS10/Car8/Dn ==
  V(t-0.83) : Inport
  0.5v : Gain  Gain=dn
  Constant : Constant  Value=dncons
  Sum : Sum  Inputs=|++
  Dn(t-0.83) : Outport
  wires:
  V(t-0.83)/1 -> 0.5v/1
  0.5v/1 -> Sum/1
  Constant/1 -> Sum/2
  Sum/1 -> Dn(t-0.83)/1

== system FS10/Car8/Translating accel to position ==
  a1t : Inport
  Discrete-Time Integrator : DiscreteIntegrator  InitialCondition=IV  InitialConditionSetting=State (most efficient)  SampleTime=-1  OutMin=0  OutMax=maxv  LimitOutput=on  UpperSaturationLimit=maxv  LowerSaturationLimit=0  ICPrevOutput=DiscIntNeverNeededParam  ICPrevScaledInput=DiscIntNeverNeededParam
  Discrete-Time Integrator1 : DiscreteIntegrator  InitialCondition=IP(8)  InitialConditionSetting=State (most efficient)  SampleTime=-1  ICPrevOutput=DiscIntNeverNeededParam  ICPrevScaledInput=DiscIntNeverNeededParam
  p1(t) : Outport
  v1t : Outport  Port=2
  wires:
  a1t/1 -> Discrete-Time Integrator/1
  Discrete-Time Integrator1/1 -> p1(t)/1
  Discrete-Time Integrator/1 -> Discrete-Time Integrator1/1, v1t/1

== system FS10/Car9/Accel Decision ==
  dx : Inport
  dv : Inport  Port=2
  Dn : Inport  Port=3
  2-D Mean : visionstatistics/2-D Mean  run=off  reset_popup=None  directionMode=Entire input  dimension=1  treatSBRowAsCol=on  roiEnable=off  roiType=Rectangles  roiPortion=Entire ROI  roiOutput=Individual statistics for each ROI  roiFlag=off  outputDataTypeStr=Inherit: Same as accumulator  outputLastDataTypeStr=Inherit: Same as accumulator  outputMin=[]  outputMax=[]  accumMode=Binary point scaling  accumWordLength=32  accumFracLength=0  accumDataTypeStr=fixdt([],32,0)  accumLastDataTypeStr=fixdt([],32,0)  roundingMode=Floor  overflowMode=off
      settings: SourceProductName=Computer Vision System Toolbox  SourceProductBaseCode=VP
  C1 : Gain  Gain=C1(9)
  Gain1 : Gain  Gain=C2(9)
  Moving Average : dspstat3/Moving Average  Method=Sliding window  SpecifyWindowLength=on  WindowLength=ave  ForgettingFactor=0.9  SimulateUsing=Code generation
  Mux1 : Mux  Inputs=2
  Saturation : Saturate  UpperLimit=maxa  LowerLimit=mina
  Sum : Sum  Inputs=|+-
  Sum1 : Sum  Inputs=|++  OutMax=[3]
  accel : Outport  OutMax=[3]  SampleTime=0.01
  wires:
  dv/1 -> C1/1
  dx/1 -> Sum/1
  Sum/1 -> Gain1/1
  C1/1 -> Sum1/1
  Gain1/1 -> Sum1/2
  Sum1/1 -> Saturation/1
  Dn/1 -> Sum/2
  Moving Average/1 -> Mux1/2
  Mux1/1 -> 2-D Mean/1
  Saturation/1 -> Moving Average/1, Mux1/1
  2-D Mean/1 -> accel/1

== system FS10/Car9/Dn ==
  V(t-0.83) : Inport
  0.5v : Gain  Gain=dn
  Constant : Constant  Value=dncons
  Sum : Sum  Inputs=|++
  Dn(t-0.83) : Outport
  wires:
  V(t-0.83)/1 -> 0.5v/1
  0.5v/1 -> Sum/1
  Constant/1 -> Sum/2
  Sum/1 -> Dn(t-0.83)/1

== system FS10/Car9/Translating accel to position ==
  a1t : Inport
  Discrete-Time Integrator : DiscreteIntegrator  InitialCondition=IV  InitialConditionSetting=State (most efficient)  SampleTime=-1  OutMin=0  OutMax=maxv  LimitOutput=on  UpperSaturationLimit=maxv  LowerSaturationLimit=0  ICPrevOutput=DiscIntNeverNeededParam  ICPrevScaledInput=DiscIntNeverNeededParam
  Discrete-Time Integrator1 : DiscreteIntegrator  InitialCondition=IP(9)  InitialConditionSetting=State (most efficient)  SampleTime=-1  ICPrevOutput=DiscIntNeverNeededParam  ICPrevScaledInput=DiscIntNeverNeededParam
  p1(t) : Outport
  v1t : Outport  Port=2
  wires:
  a1t/1 -> Discrete-Time Integrator/1
  Discrete-Time Integrator1/1 -> p1(t)/1
  Discrete-Time Integrator/1 -> Discrete-Time Integrator1/1, v1t/1

== matlab function FS10/Car1/Subsystem/low level ==
  data: vcmd input; acmd output; v input
function acmd = fcn(vcmd,v)
vdiff=vcmd-v;
if vdiff>0;
    acmd=1;
elseif vdiff<=0;
    acmd=-1;
else;
    acmd=0;
end
end

== matlab function FS10/Car1/Subsystem/V cmd ==
  data: dv input; vcmd output; dx input; v input; U input
function vcmd = fcn(dv,dx,v,U)
d=[1.5,1.0,0.5]; %deccel constant
xk0=[4.5,5.25,6.0]; %decel distance
xk0=(xk0);

xx=[0,0,0];

xx(1)=xk0(1)+(1/(2*d(1)))*(dv^2);
xx(2)=xk0(2)+(1/(2*d(2)))*(dv^2);
xx(3)=xk0(3)+(1/(2*d(3)))*(dv^2);

if dx<=xx(1);
    vcmd=0;
elseif (dx>xx(1))&&(dx<=xx(2));
    vcmd=v*(dx-xx(1))/(xx(2)-dx);
elseif (dx>xx(2))&&(dx<=xx(3));
    vcmd=v+(U-v)*(dx-xx(2))/(xx(3)-xx(2));
else
    vcmd=U;
end
end
%Needs constants for xk0,dk and U
